simulink model "vorsteuerung_mdl"  (R2013b)
settings: Solver=ode45  StartTime=0.0  StopTime=10  MaxStep=1e-3  RelTol=1e-3
libraries: cstblocks x6
settings Model: Creator=daniw  LastModifiedBy=daniw

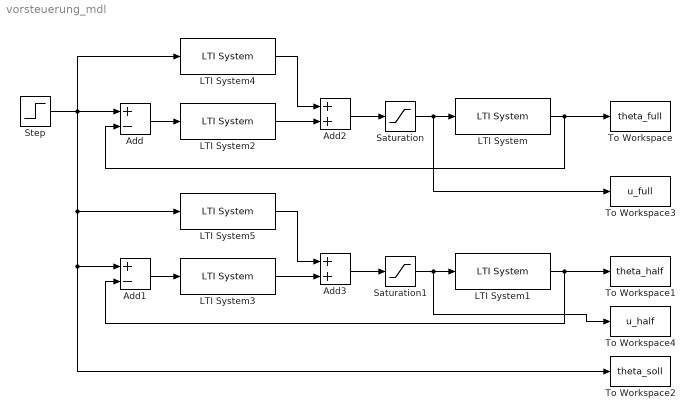
== system vorsteuerung_mdl ==
  Add : Sum  Inputs=+-
  Add1 : Sum  Inputs=+-
  Add2 : Sum
  Add3 : Sum
  LTI System : cstblocks/LTI System  sys=G1_full  IC=[]
  LTI System1 : cstblocks/LTI System  sys=G1_half  IC=[]
  LTI System2 : cstblocks/LTI System  sys=C  IC=[]
  LTI System3 : cstblocks/LTI System  sys=C  IC=[]
  LTI System4 : cstblocks/LTI System  sys=F_full  IC=[]
  LTI System5 : cstblocks/LTI System  sys=F_full  IC=[]
  Saturation : Saturate  UpperLimit=10  LowerLimit=0
  Saturation1 : Saturate  UpperLimit=10  LowerLimit=0
  Step : Step  SampleTime=0
  To Workspace : ToWorkspace  VariableName=theta_full  SampleTime=-1  SaveFormat=Structure With Time
  To Workspace1 : ToWorkspace  VariableName=theta_half  SampleTime=-1  SaveFormat=Structure With Time
  To Workspace2 : ToWorkspace  VariableName=theta_soll  SampleTime=-1  SaveFormat=Structure With Time
  To Workspace3 : ToWorkspace  VariableName=u_full  SampleTime=-1  SaveFormat=Structure With Time
  To Workspace4 : ToWorkspace  VariableName=u_half  SampleTime=-1  SaveFormat=Structure With Time
  wires:
  Step/1 -> LTI System4/1, LTI System5/1, To Workspace2/1, Add1/1, Add/1
  Add/1 -> LTI System2/1
  Add2/1 -> Saturation/1
  LTI System/1 -> To Workspace/1, Add/2
  Add1/1 -> LTI System3/1
  Add3/1 -> Saturation1/1
  LTI System1/1 -> To Workspace1/1, Add1/2
  Saturation/1 -> To Workspace3/1, LTI System/1
  Saturation1/1 -> To Workspace4/1, LTI System1/1
  LTI System2/1 -> Add2/2
  LTI System3/1 -> Add3/2
  LTI System4/1 -> Add2/1
  LTI System5/1 -> Add3/1
